simulink model "MotionObjectDetector"  (Simulink 10.0)
settings: Solver=FixedStepAuto  StartTime=0.0  StopTime=inf  RelTol=1e-3  EnableMultiTasking=on
undefined symbols (not defined in the file or in its folder): gray, Horn, hot, iut_dim, Kanade, Lucas, none, num_targets, pfactor, Rec, Schunck, SDTV, strel, target_dim, target_dim_nopyramid, videoinput
libraries: visionsinks x10, visionmorphops x7, visionanalysis x6, visionstatistics x5, visiontransforms x5, visiontextngfix x4, visionconversions x4, dspvision x3, visiongeotforms x2, visionutilities x2, imaqlib x1, visionsources x1
(part 2 of 2)

== system MotionObjectDetector/Function-Call Subsystem/Target detection and tracking/Spatial ==
  IUT : Inport
  Target : Inport  Port=2
  Enable : EnablePort  PropagateVarSize=During execution
  Normalized X-corr in spatial domain : visionstatistics/2-D Correlation  outSize=Valid  normalize=on  roundingMode=Floor  overflowMode=off  prodOutputSlope=2^-30  accumSlope=2^-30  outputSlope=2^-15
      settings: SourceProductName=Computer Vision Toolbox  SourceProductBaseCode=VP
  Out1 : Outport  InitialOutput=0
  wires:
  Target/1 -> Normalized X-corr in spatial domain/2
  IUT/1 -> Normalized X-corr in spatial domain/1
  Normalized X-corr in spatial domain/1 -> Out1/1

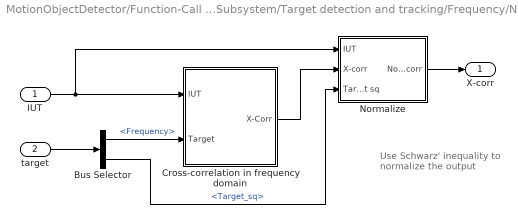
== system MotionObjectDetector/Function-Call Subsystem/Target detection and tracking/Frequency/Normalized X-corr in frequency domain ==
  note: Use Schwarz' inequality
      | to normalize the output
  IUT : Inport
  target : Inport  Port=2
  Bus Selector : BusSelector  OutputSignals=Frequency,Target_sq
  Cross-correlation in frequency domain : Subsystem
  Normalize : Subsystem
  X-corr : Outport
  wires:
  target/1 -> Bus Selector/1
  Normalize/1(Norm X-corr) -> X-corr/1
  IUT/1 -> Cross-correlation in frequency domain/1(IUT), Normalize/1(IUT)
  Cross-correlation in frequency domain/1(X-Corr) -> Normalize/2(X-corr)
  Bus Selector/1 -> Cross-correlation in frequency domain/2(Target)  "<Frequency>"
  Bus Selector/2 -> Normalize/3(Target sq)  "<Target_sq>"

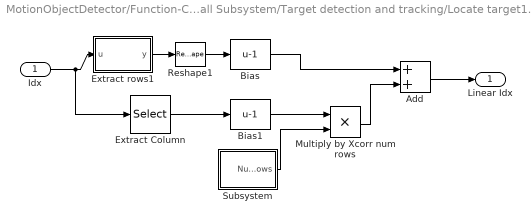
== system MotionObjectDetector/Function-Call Subsystem/Target detection and tracking/Locate target1/Convert to linear index ==
  Idx : Inport
  Add : Sum
  Bias : Bias  Bias=-1  SaturateOnIntegerOverflow=on
  Bias1 : Bias  Bias=-1  SaturateOnIntegerOverflow=on
  Extract Column : Selector  NumberOfDimensions=2  InputPortWidth=3  IndexOptions=Select all,Index vector (dialog)  Indices=[target_dim(1):iut_dim(1)],[1]  OutputSizes=1,1
  Extract rows1 : MATLAB Function  TreatAsAtomicUnit=on
  Multiply by Xcorr num rows : Product  OutDataTypeStr=uint32  RndMeth=Zero
  Reshape1 : Reshape  OutputDimensionality=Column vector (2-D)
  Subsystem : Subsystem
  Linear Idx : Outport
  wires:
  Add/1 -> Linear Idx/1
  Idx/1 -> Extract rows1/1(u), Extract Column/1
  Subsystem/1(Num Rows) -> Multiply by Xcorr num rows/2
  Extract rows1/1(y) -> Reshape1/1
  Multiply by Xcorr num rows/1 -> Add/2
  Extract Column/1 -> Bias1/1
  Bias/1 -> Add/1
  Bias1/1 -> Multiply by Xcorr num rows/1
  Reshape1/1 -> Bias/1

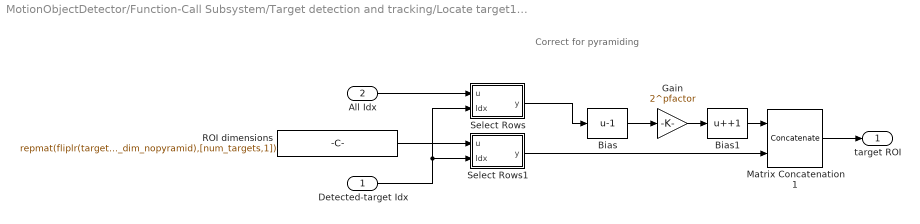
== system MotionObjectDetector/Function-Call Subsystem/Target detection and tracking/Locate target1/Create target ROIs ==
  note: Correct for
      |  pyramiding
  Detected-target Idx : Inport
  All Idx : Inport  Port=2
  Bias : Bias  Bias=-1  SaturateOnIntegerOverflow=on
  Bias1 : Bias  Bias=+1  SaturateOnIntegerOverflow=on
  Gain : Gain  Gain=2^pfactor  ParamDataTypeStr=float('single')  RndMeth=Nearest  SaturateOnIntegerOverflow=on  OutDataTypeStr=Inherit: Same as input
  Matrix Concatenation1 : Concatenate  Mode=Multidimensional array  ConcatenateDimension=2
  ROI dimensions : Constant  Value=repmat(fliplr(target_dim_nopyramid),[num_targets,1])  VectorParams1D=off  OutDataTypeStr=single
  Select Rows : MATLAB Function  TreatAsAtomicUnit=on
  Select Rows1 : MATLAB Function  TreatAsAtomicUnit=on
  target ROI : Outport
  wires:
  Detected-target Idx/1 -> Select Rows/2(Idx), Select Rows1/2(Idx)
  All Idx/1 -> Select Rows/1(u)
  Select Rows/1(y) -> Bias/1
  Matrix Concatenation1/1 -> target ROI/1
  Gain/1 -> Bias1/1
  Select Rows1/1(y) -> Matrix Concatenation1/2
  Bias/1 -> Gain/1
  Bias1/1 -> Matrix Concatenation1/1
  ROI dimensions/1 -> Select Rows1/1(u)

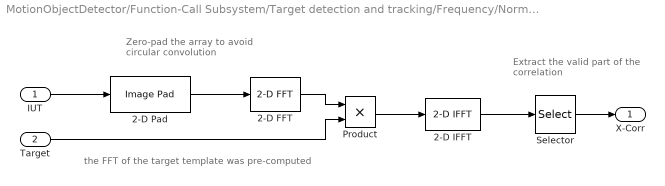
== system MotionObjectDetector/Function-Call Subsystem/Target detection and tracking/Frequency/Normalized X-corr in frequency domain/Cross-correlation in frequency domain ==
  note: Extract the valid part
      | of the correlation
  note: Zero-pad the array to avoid
      | circular convolution
  note: the FFT of the target template was pre-computed
  IUT : Inport
  Target : Inport  Port=2
  2-D FFT : visiontransforms/2-D FFT  TableOpt=NEW  TableOptActive=Speed  FFTImplementation=Auto  BitRevOrder=off  SkipNorm=off  firstCoeffLastDataTypeStr=Inherit: Same word length as input  accumLastDataTypeStr=Inherit: Same as product output  roundingMode=Floor  overflowMode=off  firstCoeffDataTypeStr=Inherit: Same word length as input  accumDataTypeStr=Inherit: Same as product output  outputMin=[]  outputMax=[]
      settings: SourceProductName=Computer Vision Toolbox  SourceProductBaseCode=VP
  2-D IFFT : visiontransforms/2-D IFFT  TableOpt=HYBRID  TableOptActive=Speed  FFTImplementation=Auto  BitRevOrder=off  cs_in=on  divideOutput=on  SkipNorm=on  firstCoeffLastDataTypeStr=Inherit: Same word length as input  accumLastDataTypeStr=Inherit: Same as product output  roundingMode=Floor  overflowMode=off  firstCoeffDataTypeStr=Inherit: Same word length as input  accumDataTypeStr=Inherit: Same as product output  outputMin=[]  outputMax=[]
      settings: SourceProductName=Computer Vision Toolbox  SourceProductBaseCode=VP
  2-D Pad : visionutilities/Image Pad  method=Constant  valSrc=Specify via dialog  value=0  spec=Output size  rowDirection=Right  outRowsMode=User-specified  rowSize=2  outColSize=2^nextpow2(iut_dim(2)+target_dim(2)+1)  colDirection=Bottom  outColsMode=User-specified  colSize=[2 3]  outRowSize=2^nextpow2(iut_dim(1)+target_dim(1)+1)  trunc_flag=None
      settings: SourceProductName=Computer Vision Toolbox  SourceProductBaseCode=VP
  Product : Product  RndMeth=Zero
  Selector : Selector  NumberOfDimensions=2  InputPortWidth=3  IndexOptions=Index vector (dialog),Index vector (dialog)  Indices=[target_dim(1):iut_dim(1)],[target_dim(2):iut_dim(2)]  OutputSizes=1,1
  X-Corr : Outport
  wires:
  2-D Pad/1 -> 2-D FFT/1
  Target/1 -> Product/2
  IUT/1 -> 2-D Pad/1
  Selector/1 -> X-Corr/1
  2-D IFFT/1 -> Selector/1
  2-D FFT/1 -> Product/1
  Product/1 -> 2-D IFFT/1

== system MotionObjectDetector/Function-Call Subsystem/Target detection and tracking/Frequency/Normalized X-corr in frequency domain/Normalize ==
  note: <a,b> matrix
  note: <a,a> scalar
  note: Schwarz' inequality:
      | -1 <= <a,b>/sqrt(<a,a>*<b,b>) <= 1
      | (here 'a' is the target and 'b' is the IUT)
  IUT : Inport
  X-corr : Inport  Port=2
  Target sq : Inport  Port=3
  <b,b> matrix : Subsystem
  Normalize : Product  Inputs=//*  SaturateOnIntegerOverflow=on  RndMeth=Zero  OutDataTypeStr=Inherit: Same as first input
  Norm X-corr : Outport
  wires:
  X-corr/1 -> Normalize/3
  Target sq/1 -> Normalize/1
  <b,b> matrix/1(<b,b>) -> Normalize/2
  Normalize/1 -> Norm X-corr/1
  IUT/1 -> <b,b> matrix/1(IUT)

== system MotionObjectDetector/Function-Call Subsystem/Target detection and tracking/Locate target1/Convert to linear index/Subsystem ==
  Selector : Selector  NumberOfDimensions=2  InputPortWidth=3  IndexOptions=Index vector (dialog),Index vector (dialog)  Indices=1,1  OutputSizes=1,1
  Xcorr dims : Constant  Value=((iut_dim-target_dim)+1)  VectorParams1D=off  OutDataTypeStr=Inherit: Inherit via back propagation
  Num Rows : Outport
  wires:
  Selector/1 -> Num Rows/1
  Xcorr dims/1 -> Selector/1

== system MotionObjectDetector/Function-Call Subsystem/Target detection and tracking/Frequency/Normalized X-corr in frequency domain/Normalize/<b,b> matrix ==
  note: use 2-D filter to
      | compute local sums
  note: Block process tiles that are the size of the target template
  IUT : Inport
  Math Function : Math  Operator=sqrt  SaturateOnIntegerOverflow=on
  Math Function1 : Math  Operator=square  SaturateOnIntegerOverflow=on
  compute local sums : visionfilter/2-D FIR Filter  separable=off  filtSrc=Specify via dialog  filterMtrx=ones(target_dim)  verticalFilter=[4 0]  horizontalFilter=[4 0]  outSize=Valid  padType=Constant  padSrc=Specify via dialog  padVal=0  method=Convolution  firstCoeffSignedness=Signed  firstCoeffLastDataTypeStr=Inherit: Same word length as input  outputSignedness=Auto  accumLastDataTypeStr=Inherit: Same as product output  roundingMode=Floor  overflowMode=off  firstCoeffDataTypeStr=Inherit: Same word length as input  firstCoeffMin=[]  firstCoeffMax=[]  accumDataTypeStr=Inherit: Same as product output  outputMin=[]  outputMax=[]
      settings: SourceProductName=Computer Vision Toolbox  SourceProductBaseCode=VP
  <b,b> : Outport
  wires:
  Math Function/1 -> <b,b>/1
  Math Function1/1 -> compute local sums/1
  IUT/1 -> Math Function1/1
  compute local sums/1 -> Math Function/1

== matlab function Display/MATLAB Function1 ==
  data: u input double; y output double size=[500,500,1]
function y = fcn(u)

if ((length(u(:,1,1)) > 1) && (length(u(1,:,1)) > 1))
    [y,~] = RedCrabMask5(u*255);
else
    y = false(500,500,1);
end

== matlab function BlobAnalysis/MATLAB Function ==
  data: image input double; roibox input double; roi output single size=[1000,1000,3]
function roi  = fcn(image, roibox)

if ((((roibox(1,2)+roibox(1,4))-1) <= length(image(:,1,1))) && (((roibox(1,1)+roibox(1,3))-1) <= length(image(1,:,1))))
    if ((roibox(1,1) ~= -1) && (roibox(1,2) ~= -1))
        roi  = image(roibox(1,2):(roibox(1,2)+roibox(1,4)-1),roibox(1,1):(roibox(1,1)+roibox(1,3)-1),:);
        
    else 
        roi = single(zeros(500,500,3));
    end
else
    roi = single(zeros(500,500,3));
end

== matlab function Function-Call Subsystem/MATLAB Function ==
  data: Image input double; redcrab input double
function fcn(Image, redcrab)

Crab = redcrab;
Scene = Image;

CrabG = rgb2gray(Crab);
SceneG = rgb2gray(Scene);

boxPoints = detectSURFFeatures(CrabG);
scenePoints = detectSURFFeatures(SceneG);
[boxFeatures, boxPoints] = extractFeatures(CrabG, boxPoints);
[sceneFeatures, scenePoints] = extractFeatures(SceneG, scenePoints);

boxPairs = matchFeatures(boxFeatures, sceneFeatures);
A = boxPairs(:, 1);
B = boxPairs(:, 2);
% matchedBoxPoints = boxPoints(A, :);
% matchedScenePoints = scenePoints(B, :);
% figure;
% showMatchedFeatures(Crab, Scene, matchedBoxPoints, ...
%     matchedScenePoints, 'montage');
% 
% [tform, inlierBoxPoints, inlierScenePoints] = ...
%     estimateGeometricTransform(matchedBoxPoints, matchedScenePoints, 'affine');
% 
% % figure;
% % showMatchedFeatures(CrabG, SceneG, inlierBoxPoints, ...
% %     inlierScenePoints, 'montage');
% % title('Matched Points (Inliers Only)');
% 
% 
% boxPolygon = [1, 1;...                           % top-left
%         size(CrabG, 2), 1;...                 % top-right
%         size(CrabG, 2), size(CrabG, 1);... % bottom-right
%         1, size(CrabG, 1);...                 % bottom-left
%         1, 1];
%     
%     
%     
% newBoxPolygon = transformPointsForward(tform, boxPolygon);
    
    
%     figure;
% imshow(Scene);
% hold on;
% line(newBoxPolygon(:, 1), newBoxPolygon(:, 2), 'Color', 'y');
% title('Detected Box');


% matchedCrabPoints = RedCrabPoints(RedCrabPairs(:,1),:);

% matchedImagePoints = ROIPoints(RedCrabPairs(:,2),:);

% figure;
% showMatchedFeatures(redcrabGray, ImageGray, matchedCrabPoints, matchedImagePoints, 'montage');

== matlab function Function-Call Subsystem/MATLAB Function1 ==
  data: Image input double; redcrab input double
function fcn(Image, redcrab)

redcrabGray = rgb2gray(redcrab);
ImageGray = rgb2gray(Image);
RedCrabPoints = detectSURFFeatures(redcrabGray);

[RedCrabFeatures, RedCrabPoints] = extractFeatures(redcrabGray, RedCrabPoints);

ROIPoints = detectSURFFeatures(ImageGray);
[ROIFeatures, ROIPoints] = extractFeatures(ImageGray, ROIPoints);


RedCrabPairs = matchFeatures(RedCrabFeatures, ROIFeatures);

% matchedCrabPoints = RedCrabPoints(RedCrabPairs(:,1),:);

% matchedImagePoints = ROIPoints(RedCrabPairs(:,2),:);

% figure;
% showMatchedFeatures(redcrabGray, ImageGray, matchedCrabPoints, matchedImagePoints, 'montage');

== matlab function Function-Call Subsystem/Target detection and tracking/Locate target1/Convert to linear index/Extract rows1 ==
  data: u input double; y output double
function y = fcn(u)
%#codegen
l = size(u); 
y = u(:,l(2));

== matlab function Function-Call Subsystem/Target detection and tracking/Locate target1/Create target ROIs/Select Rows ==
  data: u input double; y output double; Idx input double
function y = fcn(u, Idx)
%#codegen

y = u;
y(~Idx,:)=0;

== matlab function Function-Call Subsystem/Target detection and tracking/Locate target1/Create target ROIs/Select Rows1 ==
  data: u input double; y output double; Idx input double
function y = fcn(u, Idx)
%#codegen

y = u;
y(~Idx,:)=0;
